simulink model "lab2SimulinkControl"  (R2021b)
settings: Solver=VariableStepAuto  StartTime=0.0  StopTime=15  RelTol=1e-3
undefined symbols (not defined in the file): kd, ki, kp, r1, r2, r3, TFden, TFnum
libraries: fl_lib x9, nesl_utility x3
settings Model: Creator=nicol  LastModifiedBy=nicol

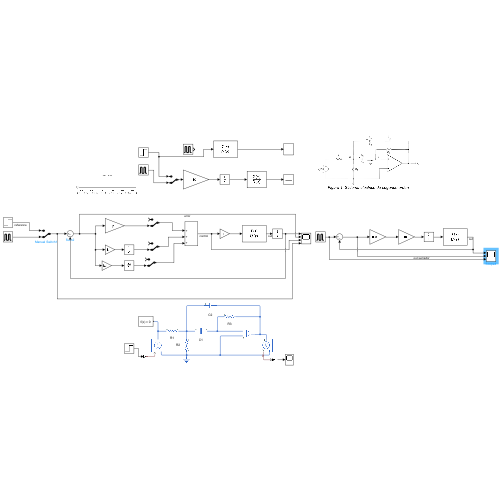
[thumbnail: Simulink's stored preview of the top-level diagram]
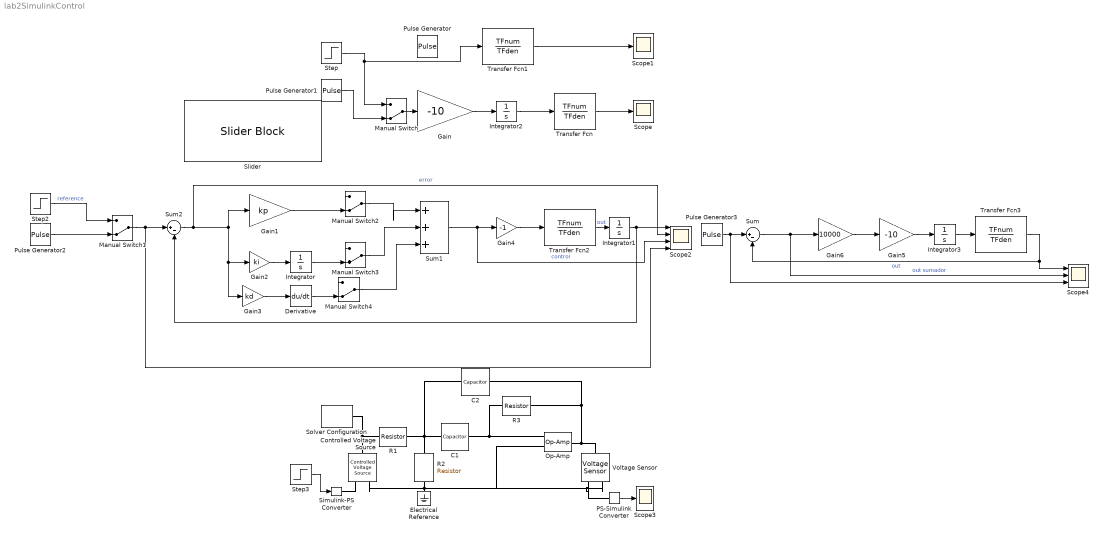
== system lab2SimulinkControl ==
  C1 : fl_lib/Electrical/Electrical Elements/Capacitor  c=c1 F  r=1e-6 Ohm  g=0 1/Ohm  i_specify=off  i_priority=None  i=0 A  i_nominal_specify=off  i_nominal_unit=A  i_nominal_value=1  v_specify=off  v_priority=None  v=0 V  v_nominal_specify=off  v_nominal_unit=V  v_nominal_value=1  vc_specify=off  vc_priority=High  vc=0 V  vc_nominal_specify=off  vc_nominal_unit=V  vc_nominal_value=1
  C2 : fl_lib/Electrical/Electrical Elements/Capacitor  c=c2 F  r=1e-6 Ohm  g=0 1/Ohm  i_specify=off  i_priority=None  i=0 A  i_nominal_specify=off  i_nominal_unit=A  i_nominal_value=1  v_specify=off  v_priority=None  v=0 V  v_nominal_specify=off  v_nominal_unit=V  v_nominal_value=1  vc_specify=off  vc_priority=High  vc=0 V  vc_nominal_specify=off  vc_nominal_unit=V  vc_nominal_value=1
  Controlled Voltage Source : fl_lib/Electrical/Electrical Sources/Controlled Voltage Source
  Derivative : Derivative
  Electrical Reference : fl_lib/Electrical/Electrical Elements/Electrical Reference
  Gain : Gain  Gain=-10
  Gain1 : Gain  Gain=kp
  Gain2 : Gain  Gain=ki
  Gain3 : Gain  Gain=kd
  Gain4 : Gain  Gain=-1
  Gain5 : Gain  Gain=-10
  Gain6 : Gain  Gain=10000
  Integrator{,1..3} (4 alike) : Integrator
  Manual Switch{,1..4} (5 alike) : ManualSwitch  CurrentSetting=0
  Op-Amp : fl_lib/Electrical/Electrical Elements/Op-Amp  outI_specify=off  outI_priority=None  outI=0 A  outI_nominal_specify=off  outI_nominal_unit=A  outI_nominal_value=1
  PS-Simulink Converter : nesl_utility/PS-Simulink Converter  PhysicalDomain=network_engine_domain  SubClassName=ps_output  LeftPortType=input  RightPortType=output  PseudoPeriodic=off  Frequencies=[]  Unit=inherit  AffineConversion=off
      settings: SourceProductBaseCode=PW,SS
  Pulse Generator : DiscretePulseGenerator  PulseType=Time based  Amplitude=5  Period=1  PulseWidth=5
  Pulse Generator1 : DiscretePulseGenerator  PulseType=Time based  Amplitude=7  PulseWidth=5
  Pulse Generator2 : DiscretePulseGenerator  PulseType=Time based  Amplitude=5  Period=5  PulseWidth=50
  Pulse Generator3 : DiscretePulseGenerator  PulseType=Time based  Amplitude=5  Period=20  PulseWidth=50
  R1 : fl_lib/Electrical/Electrical Elements/Resistor  R=r1 Ohm  i_specify=off  i_priority=None  i=0 A  i_nominal_specify=off  i_nominal_unit=A  i_nominal_value=1  v_specify=off  v_priority=None  v=0 V  v_nominal_specify=off  v_nominal_unit=V  v_nominal_value=1
  R2 : fl_lib/Electrical/Electrical Elements/Resistor  R=r2 Ohm  i_specify=off  i_priority=None  i=0 A  i_nominal_specify=off  i_nominal_unit=A  i_nominal_value=1  v_specify=off  v_priority=None  v=0 V  v_nominal_specify=off  v_nominal_unit=V  v_nominal_value=1
  R3 : fl_lib/Electrical/Electrical Elements/Resistor  R=r3 Ohm  i_specify=off  i_priority=None  i=0 A  i_nominal_specify=off  i_nominal_unit=A  i_nominal_value=1  v_specify=off  v_priority=None  v=0 V  v_nominal_specify=off  v_nominal_unit=V  v_nominal_value=1
  Scope : Scope
  Scope1 : Scope
  Scope2 : Scope  NumInputPorts=4
  Scope3 : Scope
  Scope4 : Scope  NumInputPorts=3
  Simulink-PS Converter : nesl_utility/Simulink-PS Converter  PhysicalDomain=network_engine_domain  SubClassName=ps_input  LeftPortType=input  RightPortType=output  PseudoPeriodic=off  Frequencies=[]  NoiseDistribution=none  NoiseParameters=[]  Unit=1  AffineConversion=off  FilteringAndDerivatives=provide  SimscapeFilterOrder=1  InputFilterTimeConstant=0.001  UdotUserProvided=0
      settings: SourceProductBaseCode=PW,SS
  Slider : SliderBlock  ScaleMin=2.5  ScaleMax=3
  Solver Configuration : nesl_utility/Solver Configuration  PhysicalDomain=network_engine_domain  SubClassName=solver  LeftPortType=input  RightPortType=generic  Tones=[]  Harmonics=[]  SimulateNoise=off  Profile=off  UseLocalSampling=off  EnableSwitchedLinearOptims=on  FrequencyDomain=off  UseCCode=off  RelTol=0.001  AbsTol=1e-06  MinStep=1e-09  ToWorkspace=off  RevertToSquareIcSolve=off  NumHomotopyIterations=100  PhasorMode=off  PhasorModeNumHarmonics=1  DoDC=off  ResidualTolerance=1e-09  UseLocalSolver=off  LocalSolverChoice=NE_BACKWARD_EULER_ADVANCER  LocalSolverSampleTime=0.001  DoFixedCost=off  MaxNonlinIter=3  MaxModeIter=2  ComputeImpulses=off  ImpulseIterations=2  LinearAlgebra=auto  EquationFormulation=NE_TIME_EF  DelaysMemoryBudget=1024  AutomaticFiltering=on  FilteringTimeConstant=0.001  PartitionStorageMethod=AS_NEEDED  PartitionMemoryBudget=1024  PartitionMethod=ROBUST
      settings: SourceProductBaseCode=PW,SS
  Step : Step  Time=0  After=5  SampleTime=0
  Step2 : Step  Time=0  After=5  SampleTime=0
  Step3 : Step  Time=0  SampleTime=0
  Sum : Sum  Inputs=|+-
  Sum1 : Sum  Inputs=|+++
  Sum2 : Sum  Inputs=|+-
  Transfer Fcn{,1..3} (4 alike) : TransferFcn  Numerator=TFnum  Denominator=TFden
  Voltage Sensor : fl_lib/Electrical/Electrical Sensors/Voltage Sensor
  wires:
  Transfer Fcn/1 -> Scope/1
  Gain/1 -> Integrator2/1
  Transfer Fcn1/1 -> Scope1/1
  Step3/1 -> Simulink-PS Converter/1
  PS-Simulink Converter/1 -> Scope3/1
  Gain2/1 -> Integrator/1
  Sum2/1 -> Scope2/2, Gain1/1, Gain3/1, Gain2/1  "error"
  Gain3/1 -> Derivative/1
  Sum1/1 -> Scope2/3, Gain4/1  "control"
  Integrator2/1 -> Transfer Fcn/1
  Gain4/1 -> Transfer Fcn2/1
  Transfer Fcn2/1 -> Integrator1/1  "out"
  Integrator1/1 -> Sum2/2, Scope2/1
  Gain5/1 -> Integrator3/1
  Transfer Fcn3/1 -> Sum/2, Scope4/1  "out"
  Integrator3/1 -> Transfer Fcn3/1
  Pulse Generator3/1 -> Scope4/3, Sum/1
  Sum/1 -> Scope4/2, Gain6/1  "out sumador"
  Manual Switch/1 -> Gain/1
  Step/1 -> Transfer Fcn1/1, Manual Switch/1
  Pulse Generator1/1 -> Manual Switch/2
  Manual Switch1/1 -> Scope2/4, Sum2/1
  Pulse Generator2/1 -> Manual Switch1/2
  Step2/1 -> Manual Switch1/1  "reference"
  Manual Switch2/1 -> Sum1/1
  Gain1/1 -> Manual Switch2/2
  Manual Switch3/1 -> Sum1/2
  Integrator/1 -> Manual Switch3/2
  Derivative/1 -> Manual Switch4/2
  Manual Switch4/1 -> Sum1/3
  Gain6/1 -> Gain5/1
  connections:
  Op-Amp/LConn2 -- R3/LConn1 -- C1/RConn1
  R3/RConn1 -- Voltage Sensor/LConn1 -- Op-Amp/RConn1 -- C2/RConn1
  Electrical Reference/LConn1 -- Voltage Sensor/RConn2 -- Op-Amp/LConn1 -- Controlled Voltage Source/RConn2 -- R2/RConn1
  R2/LConn1 -- C2/LConn1 -- R1/RConn1 -- C1/LConn1
  Controlled Voltage Source/LConn1 -- Solver Configuration/RConn1 -- R1/LConn1
  Controlled Voltage Source/RConn1 -- Simulink-PS Converter/RConn1
  Voltage Sensor/RConn1 -- PS-Simulink Converter/LConn1
